simulink model "float_mch_Sample_HardThreshold"  (R2020a)
settings: Solver=VariableStepAuto  StartTime=0  StopTime=30  RelTol=1e-3
model workspace (MAT data in the model file):
  a = 0
libraries: dspfdesign x2, dspswit3 x1, simulink x1
settings Model: SimulationMode=accelerator  Creator=sbuccelli  LastModifiedBy=diflo

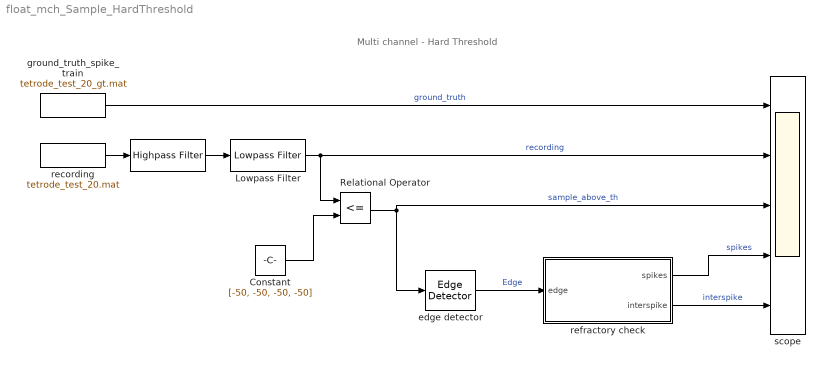
== system float_mch_Sample_HardThreshold ==
  note: Multi channel - Hard Threshold
  " " : dspfdesign/Highpass Filter  FilterType=IIR  DesignForMinimumOrder=on  FilterOrder=50  StopbandFrequency=1  PassbandFrequency=300  StopbandAttenuation=80  PassbandRipple=0.1  InheritSampleRate=off  SampleRate=fs  SimulateUsing=Interpreted execution  roundingMode=Floor  coeffsDataTypeStr=fixdt(1,16)
  Constant : Constant  Value=[-50, -50, -50, -50]
  Lowpass Filter : dspfdesign/Lowpass Filter  FilterType=IIR  DesignForMinimumOrder=on  FilterOrder=3  PassbandFrequency=3500  StopbandFrequency=8500  PassbandRipple=0.1  StopbandAttenuation=80  InheritSampleRate=off  SampleRate=fs  SimulateUsing=Interpreted execution  roundingMode=Floor  coeffsDataTypeStr=fixdt(1,16)
  Relational Operator : RelationalOperator  Operator=<=  OutDataTypeStr=boolean  RndMeth=Simplest
  "edge detector " : dspswit3/Edge Detector  InputProcessing=Columns as channels (frame based)
      settings: SourceProductBaseCode=DS
  ground_truth_spike_train : FromFile  FileName=tetrode_test_20_gt.mat  SampleTime=1/30000
  recording : FromFile  FileName=tetrode_test_20.mat  SampleTime=1/30000
  refractory check : Subsystem
  scope : Scope  NumInputPorts=5
  wires:
  Relational Operator/1 -> scope/3, "edge detector "/1  "sample_above_th"
  "edge detector "/1 -> refractory check/1("edge  ")  "Edge"
  refractory check/2(interspike) -> scope/5  "interspike"
  refractory check/1(spikes) -> scope/4  "spikes"
  Constant/1 -> Relational Operator/2
  recording/1 -> " "/1
  ground_truth_spike_train/1 -> scope/1  "ground_truth"
  " "/1 -> Lowpass Filter/1
  Lowpass Filter/1 -> scope/2, Relational Operator/1  "recording"

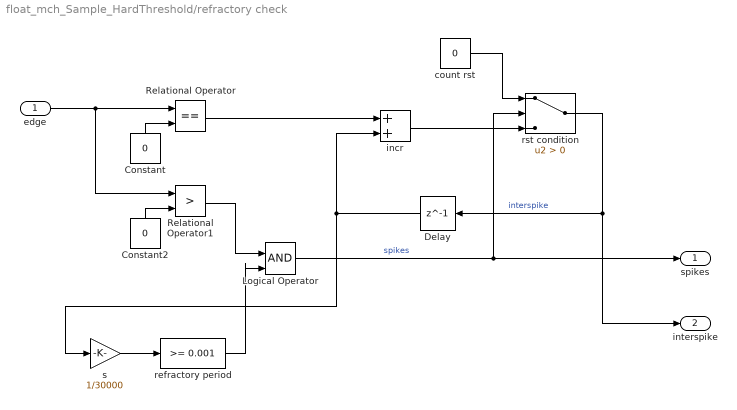
== system float_mch_Sample_HardThreshold/refractory check ==
  "edge  " : Inport
  Constant : Constant  Value=0
  Constant2 : Constant  Value=0
  Delay : Delay  DelayLength=1  InitialCondition=1
  Logical Operator : Logic  IconShape=distinctive  AllPortsSameDT=off  OutDataTypeStr=boolean
  Relational Operator : RelationalOperator  Operator===  OutDataTypeStr=boolean  RndMeth=Simplest
  Relational Operator1 : RelationalOperator  Operator=>  OutDataTypeStr=boolean  RndMeth=Simplest
  count rst : Constant  Value=0
  incr : Sum  AccumDataTypeStr=double
  refractory period : simulink/Logic and Bit Operations/Compare To Constant  relop=>=  const=0.001  OutDataTypeStr=boolean
  rst condition : Switch  Criteria=u2 > Threshold  OutDataTypeStr=double
  s : Gain  Gain=1/30000
  spikes : Outport
  interspike : Outport  Port=2
  wires:
  count rst/1 -> rst condition/1
  Constant/1 -> Relational Operator/2
  Constant2/1 -> Relational Operator1/2
  Relational Operator1/1 -> Logical Operator/1
  refractory period/1 -> Logical Operator/2
  Logical Operator/1 -> spikes/1, rst condition/2  "spikes"
  incr/1 -> rst condition/3
  rst condition/1 -> interspike/1, Delay/1  "interspike"
  Delay/1 -> s/1, incr/2
  Relational Operator/1 -> incr/1
  "edge  "/1 -> Relational Operator1/1, Relational Operator/1
  s/1 -> refractory period/1
